simulink model "mppt"  (R2016b)
settings: Solver=VariableStepAuto  StartTime=0.0  StopTime=10.0  RelTol=1e-3
settings Model: Creator=root  LastModifiedBy=root

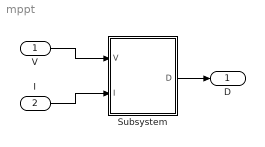
== system mppt ==
  V : Inport
  I : Inport  Port=2
  Subsystem : Subsystem
  "D " : Outport
  wires:
  V/1 -> Subsystem/1(V)
  I/1 -> Subsystem/2(I)
  Subsystem/1("D ") -> "D "/1

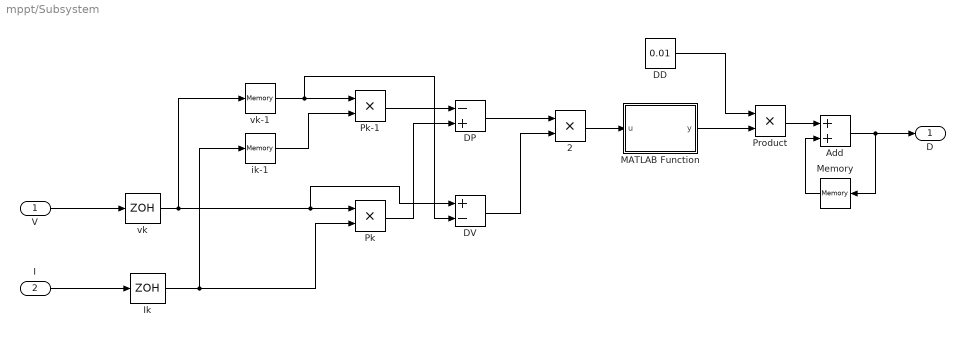
== system mppt/Subsystem ==
  V : Inport
  I : Inport  Port=2
  2 : Product
  Add : Sum
  DD : Constant  Value=0.01
  DP : Sum  Inputs=-+
  DV : Sum  Inputs=+-
  Ik : ZeroOrderHold  SampleTime=1e-3
  MATLAB Function : MATLAB Function  TreatAsAtomicUnit=on
  Memory : Memory
  Pk : Product
  Pk-1 : Product
  Product : Product
  ik-1 : Memory
  vk : ZeroOrderHold  SampleTime=1e-3
  vk-1 : Memory
  "D " : Outport
  wires:
  Memory/1 -> Add/2
  Add/1 -> "D "/1, Memory/1
  DD/1 -> Product/1
  Product/1 -> Add/1
  MATLAB Function/1(y) -> Product/2
  ik-1/1 -> Pk-1/2
  V/1 -> vk/1
  I/1 -> Ik/1
  Ik/1 -> ik-1/1, Pk/2
  vk/1 -> vk-1/1, DV/1, Pk/1
  Pk-1/1 -> DP/1
  Pk/1 -> DP/2
  DP/1 -> 2/1
  DV/1 -> 2/2
  2/1 -> MATLAB Function/1(u)
  vk-1/1 -> DV/2, Pk-1/1

== matlab function mppt/Subsystem/MATLAB Function ==
  data: u input; y output
function y = fcn(u)
y=0;
if(u==0)
    y=0;
end
if(u>0)
    y=-1;
end
if(u<0)
    y=1;
end
